simulink model "MultiObjectTracking"  (R2022a)
settings: Solver=VariableStepAuto  StartTime=0.0  StopTime=10.0  RelTol=1e-3
libraries: drivingscenarioandsensors x2, motalgorithmslib x1
settings Model: Creator=mciti  LastModifiedBy=mciti

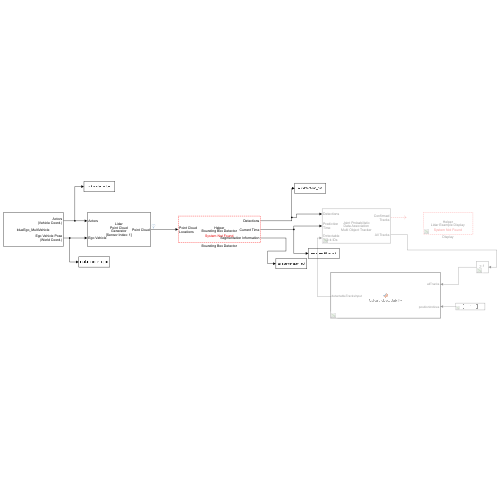
[thumbnail: Simulink's stored preview of the top-level diagram]
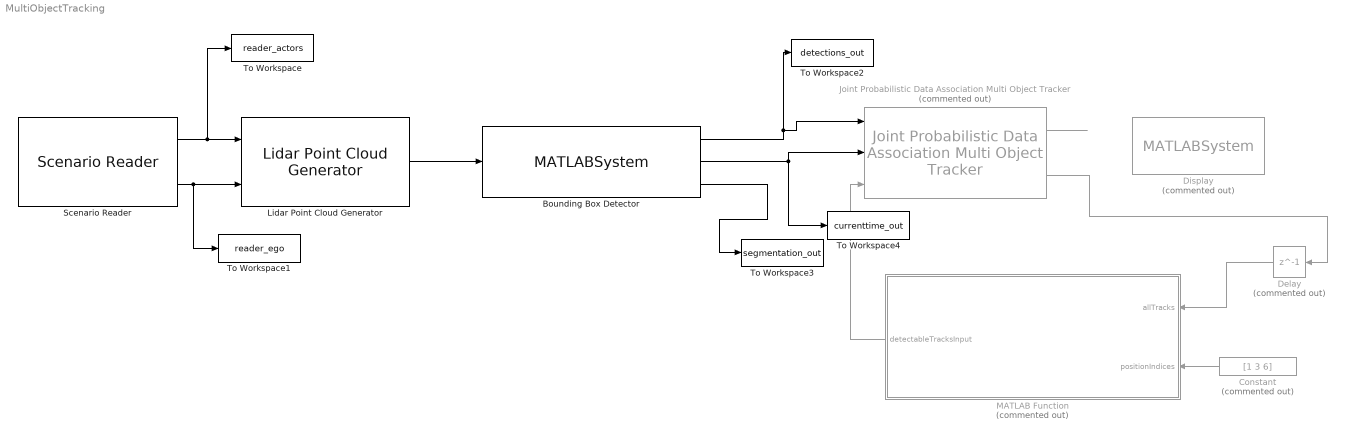
== system MultiObjectTracking ==
  Bounding Box Detector : MATLABSystem  System=HelperBoundingBoxDetectorBlock  DetectionBusName=detectionBus  SegmentationBusName=segmentationBus  NumLidarPoints=55000  XLimits=[ -70, 70 ]  YLimits=[ -6, 6 ]  ZLimits=[ -2, 10 ]  GroundMaxDistance=0.3  GroundReferenceVector=[ 0, 0, 1 ]  GroundMaxAngularDistance=5  SegmentationMinDistance=1.6  MinDetectionsPerCluster=2  MaxZDistanceCluster=3  MinZDistanceCluster=-3  EgoVehicleRadius=2  MeasurementNoise=blkdiag( eye( 3 ), 10, eye( 3 ) )  MeasurementParameters=struct.empty( 0, 1 )  SimulateUsing=Code generation
      mask Type: HelperBoundingBoxDetectorBlock
      mask Display:
      | disp(['Helper' char(10) 'Bounding Box Detector']);
      | port_label('input',1,['Point Cloud' char(10) 'Locations']);
      | port_label('output',1,'Detections');
      | port_label('output',2,'Current Time');
      | port_label('output',3,'Segmentation Information');
  Constant : Constant  Commented=on  Value=[1 3 6]
  Delay : Delay  Commented=on  DelayLength=1
  Display : MATLABSystem  Commented=on  System=HelperLidarExampleDisplayBlock  LidarDataReaderBlockName=Lidar Point Cloud Generator  DetectorBlockName=Bounding Box Detector  TrackerBlockName=Joint Probabilistic Data Association Multi Object Tracker  PositionIndex=[ 1, 3, 6 ]  VelocityIndex=[ 2, 4, 7 ]  DimensionIndex=[ 9, 11, 13 ]  YawIndex=8  RecordGIF=false  SimulateUsing=Interpreted execution
      mask Type: HelperLidarExampleDisplayBlock
      mask Display: disp(['Helper' char(10) 'Lidar Example Display']);
  Joint Probabilistic Data Association Multi Object Tracker : motalgorithmslib/Joint Probabilistic Data Association Multi Object Tracker  Commented=on  TrackerIndex=uint32( 0 )  FilterInitializationFcn=initcvekf  MaxNumEvents=inf  EventGenerationFcn=jpdaEvents  MaxNumTracks=100  MaxNumSensors=20  TimeTolerance=1e-5  OOSMHandling=Terminate  MaxNumOOSMSteps=3  StateParametersSimulink=struct  HasStateParametersInput=off  EnableMemoryManagement=off  SimulateUsing=Interpreted execution  AssignmentThreshold=[ 1, Inf ] * 30.0  InitializationThreshold=0  DetectionProbability=0.9  ClutterDensity=1e-6  TrackLogic=History  pHistoryConfThreshold=[ 2, 3 ]  pHistoryDelThreshold=[ 5, 5 ]  pIntegratedConfThreshold=0.95  pIntegratedDelThreshold=0.1  HitMissThreshold=0.2  NewTargetDensity=1e-5  DeathRate=0.01  TimeInputSource=Input port  HasCostMatrixInput=off  HasDetectableTrackIDsInput=on  TentativeTracksOutputPort=off  AllTracksOutputPort=on  InfoOutputPort=off  BusNameSource=Auto  BusName=BusTrackerJPDA  BusName2Source=Auto  BusName2=BusTrackerInfo  MaxNumDetectionsPerSensor=100  MaxNumDetectionsPerCluster=5  MaxNumTracksPerCluster=5  ClusterViolationHandling=Split and warn
      settings: SourceProductBaseCode=TF
  Lidar Point Cloud Generator : drivingscenarioandsensors/Lidar Point Cloud Generator  SensorIndex=1  UpdateInterval=0.1  SensorLocation=[1.5 0]  Height=1.6  Yaw=0  Pitch=0  Roll=0  DetectionCoordinates=Ego Cartesian  HasEgoVehicle=on  EgoVehicleActorID=1  HasRoadsInputPort=on  ActorProfilesSource=From Scenario Reader block  ActorProfilesVariableName=actor_profiles  MaxRange=120  RangeAccuracy=0.002  AzimuthResolution=0.16  ElevationResolution=1.25  AzimuthLimits=[ -180, 180 ]  ElevationLimits=[ -20, 20 ]  HasNoise=on
      settings: SourceProductBaseCode=DR
  MATLAB Function : MATLAB Function  Commented=on  TreatAsAtomicUnit=on
  Scenario Reader : drivingscenarioandsensors/Scenario Reader  ScenarioSource=From file  ScenarioFileName=C:\Users\mciti\Documents\Projects\matlab_ws\ADAS_project\withSimulink\scenarios\blueEgo_MultiVehicle.mat  ScenarioVariableName=scenario  OutputCoordinateSystem=Vehicle coordinates  EgoVehicleSource=Scenario  EgoVehicleActorID=1  OrientVehiclesOnRoad=off  OutputEgoVehiclePose=on  OutputEgoVehicleState=off  SampleTime=0.1  LaneBoundaryOutput=None  LaneBoundaryDistance=0:0.5:9.5  LaneBoundaryLocation=Center of lane markings  BusNameSource=Auto  BusName=BusActors  BusNumActorsSource=Scenario  BusNumActors=100  BusName2Source=Auto  BusName2=BusLaneBoundaries  BusNumLaneBoundariesSource=Scenario  BusNumLaneBoundaries=10  BusName3Source=Auto  BusName3=BusEgoActor  BusName4Source=Auto  BusName4=BusEgoState  ShowCoordinateLabels=on  SimulateUsing=Interpreted execution
  To Workspace : ToWorkspace  VariableName=reader_actors  SaveFormat=Timeseries  SampleTime=-1
  To Workspace1 : ToWorkspace  VariableName=reader_ego  SaveFormat=Timeseries  SampleTime=-1
  To Workspace2 : ToWorkspace  VariableName=detections_out  SaveFormat=Timeseries  SampleTime=-1
  To Workspace3 : ToWorkspace  VariableName=segmentation_out  SaveFormat=Timeseries  SampleTime=-1
  To Workspace4 : ToWorkspace  VariableName=currenttime_out  SaveFormat=Timeseries  SampleTime=-1
  wires:
  Scenario Reader/1 -> To Workspace/1, Lidar Point Cloud Generator/1
  Scenario Reader/2 -> To Workspace1/1, Lidar Point Cloud Generator/2
  Bounding Box Detector/2 -> Joint Probabilistic Data Association Multi Object Tracker/2, To Workspace4/1
  Bounding Box Detector/1 -> To Workspace2/1, Joint Probabilistic Data Association Multi Object Tracker/1
  Joint Probabilistic Data Association Multi Object Tracker/1 -> ?
  Joint Probabilistic Data Association Multi Object Tracker/2 -> Delay/1
  Delay/1 -> MATLAB Function/1(allTracks)
  MATLAB Function/1(detectableTracksInput) -> Joint Probabilistic Data Association Multi Object Tracker/3
  Constant/1 -> MATLAB Function/2(positionIndices)
  Bounding Box Detector/3 -> To Workspace3/1
  Lidar Point Cloud Generator/1 -> Bounding Box Detector/1

== matlab function MultiObjectTracking/MATLAB Function ==
  data: allTracks input; detectableTracksInput output; positionIndices input
function detectableTracksInput = CalculateDetectability(allTracks, positionIndices)
% This function calculates the probability of detection for each track. The
% helperCalcDetectability function is used to compute the probability after
% extracting the tracks from the bus.
tracks = allTracks.Tracks(1:allTracks.NumTracks);
detectableTracksInput = helperCalcDetectability(tracks, positionIndices);
end
